simulink model "Reduce_Block_Diagram_TF_1"  (R2024a)
settings: Solver=VariableStepAuto  StartTime=0.0  StopTime=10  RelTol=1e-3
undefined symbols (not defined in the file or in its folder): TF_den, TF_num

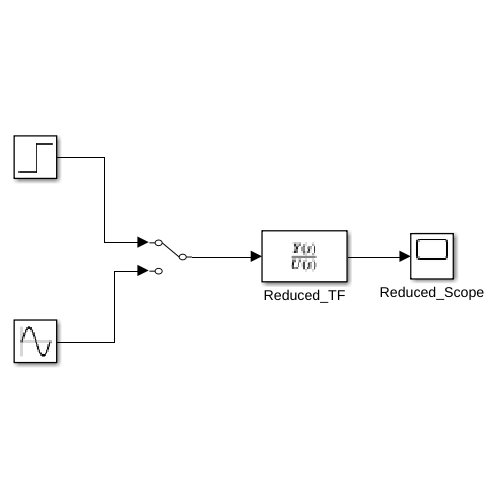
[thumbnail: Simulink's stored preview of the top-level diagram]
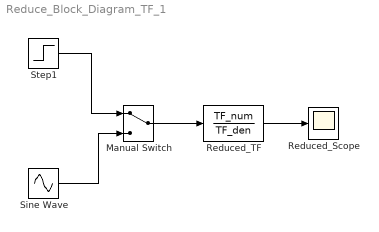
== system Reduce_Block_Diagram_TF_1 ==
  Manual Switch : ManualSwitch
  Reduced_Scope : Scope
  Reduced_TF : TransferFcn  Numerator=TF_num  Denominator=TF_den
  Sine Wave : Sin  SampleTime=0
  Step1 : Step  Time=0  SampleTime=0
  wires:
  Reduced_TF/1 -> Reduced_Scope/1
  Step1/1 -> Manual Switch/1
  Sine Wave/1 -> Manual Switch/2
  Manual Switch/1 -> Reduced_TF/1
